simulink model "AEROATCSS"  (R2024b)
settings: Solver=ode45  StartTime=0.0  StopTime=10000  MaxStep=0.25  RelTol=1e-3
PreLoadFcn:
  | initialize_model_data;
  | appdesignparameteraeroatcss_exported_last1;
model workspace (MAT data in the model file):
  AZ_Sep = Simulink.Parameter
  AZ_Sep.Complexity = 'real'
  AZ_Sep.Dimensions = [0 0]
  AZ_Sep.DataType = 'auto'
  BwPw = Simulink.Parameter
  BwPw.Complexity = 'real'
  BwPw.Dimensions = [0 0]
  BwPw.DataType = 'auto'
  E = Simulink.Parameter
  E.Complexity = 'real'
  E.Dimensions = [0 0]
  E.DataType = 'auto'
  EL_Sep = Simulink.Parameter
  EL_Sep.Complexity = 'real'
  EL_Sep.Dimensions = [0 0]
  EL_Sep.DataType = 'auto'
  Lambda = Simulink.Parameter
  Lambda.Complexity = 'real'
  Lambda.Dimensions = [0 0]
  Lambda.DataType = 'auto'
  Loss = Simulink.Parameter
  Loss.Complexity = 'real'
  Loss.Dimensions = [0 0]
  Loss.DataType = 'auto'
  Noise = Simulink.Parameter
  Noise.Complexity = 'real'
  Noise.Dimensions = [0 0]
  Noise.DataType = 'auto'
  Pt = Simulink.Parameter
  Pt.Complexity = 'real'
  Pt.Dimensions = [0 0]
  Pt.DataType = 'auto'
  Rres = Simulink.Parameter
  Rres.Complexity = 'real'
  Rres.Dimensions = [0 0]
  Rres.DataType = 'auto'
  SNR = Simulink.Parameter
  SNR.Complexity = 'real'
  SNR.Dimensions = [0 0]
  SNR.DataType = 'auto'
  Temp = Simulink.Parameter
  Temp.Complexity = 'real'
  Temp.Dimensions = [0 0]
  Temp.DataType = 'auto'
  rainfall = Simulink.Parameter
  rainfall.Complexity = 'real'
  rainfall.Dimensions = [0 0]
  rainfall.DataType = 'auto'
values from neighbouring files (symbols this model uses):
  lambda_bp = [0.057, 0.075, 0.1, 0.15, 0.3]    [initialize_model_data.m]
  rainfall_bp = [0.0, 0.25, 1, 4, 16]    [initialize_model_data.m]
  sigma_table = [ ... (first row only)    [initialize_model_data.m]
settings Model: Creator=Sangam  LastModifiedBy=Sangam
settings DataIOCC: SaveFormat=Array  SaveOutput=off  SignalLogging=off  SaveTime=off  ReturnWorkspaceOutputs=off
settings DebuggingCC: MultiTaskCondExecSysMsg=none
settings ModelReferenceCC: EnableRefExpFcnMdlSchedulingChecks=on  PropagateSignalLabelsOutOfModel=off

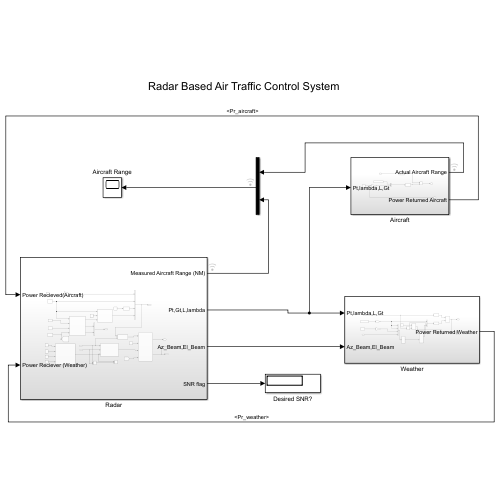
[thumbnail: Simulink's stored preview of the top-level diagram]
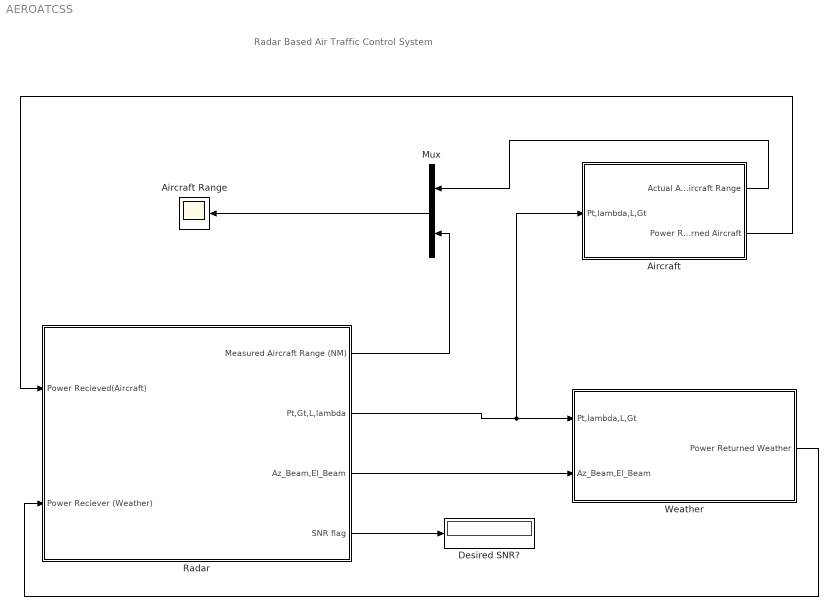
== system AEROATCSS ==
  note: Radar Based Air Traffic Control System
  Aircraft : Subsystem
  Aircraft Range : Scope
  Desired SNR? : Display
  Mux : Mux  Inputs=2
  Radar : Subsystem
  Weather : Subsystem
  wires:
  Radar/4(SNR flag) -> Desired SNR?/1
  Radar/1(Measured Aircraft Range (NM)) -> Mux/2
  Radar/2(Pt,Gt,L,lambda) -> Aircraft/1(Pt,lambda,L,Gt), Weather/1(Pt,lambda,L,Gt)
  Radar/3(Az_Beam,El_Beam) -> Weather/2(Az_Beam,El_Beam)
  Weather/1(Power Returned Weather) -> Radar/2("Power Reciever (Weather) ")
  Aircraft/1(Actual Aircraft Range) -> Mux/1
  Mux/1 -> Aircraft Range/1
  Aircraft/2(Power Returned Aircraft) -> Radar/1(Power Recieved(Aircraft))

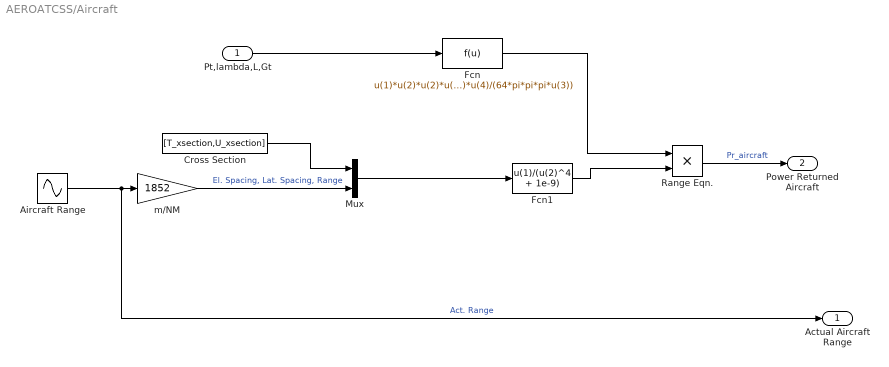
== system AEROATCSS/Aircraft ==
  Pt,lambda,L,Gt : Inport
  Aircraft Range : Sin  Amplitude=25  Bias=35  Frequency=0.0025  SampleTime=0
  Cross Section : FromWorkspace  VariableName=[T_xsection,U_xsection]  Interpolate=off  ZeroCross=off  OutputAfterFinalValue=Holding final value
  Fcn : Fcn  Expr=u(1)*u(2)*u(2)*u(4)*u(4)/(64*pi*pi*pi*u(3))
  Fcn1 : Fcn  Expr=u(1)/(u(2)^4 + 1e-9)
  Mux : Mux  Inputs=2
  Range Eqn. : Product  InputSameDT=on  RndMeth=Zero  SaturateOnIntegerOverflow=on  OutDataTypeStr=Inherit: Same as first input
  m/NM : Gain  Gain=1852
  Actual Aircraft Range : Outport
  Power Returned Aircraft : Outport  Port=2
  wires:
  Fcn1/1 -> Range Eqn./2
  Mux/1 -> Fcn1/1
  Aircraft Range/1 -> Actual Aircraft Range/1, m/NM/1  "Act. Range"
  m/NM/1 -> Mux/2  "El. Spacing, Lat. Spacing, Range"
  Pt,lambda,L,Gt/1 -> Fcn/1
  Range Eqn./1 -> Power Returned Aircraft/1  "Pr_aircraft"
  Cross Section/1 -> Mux/1
  Fcn/1 -> Range Eqn./1

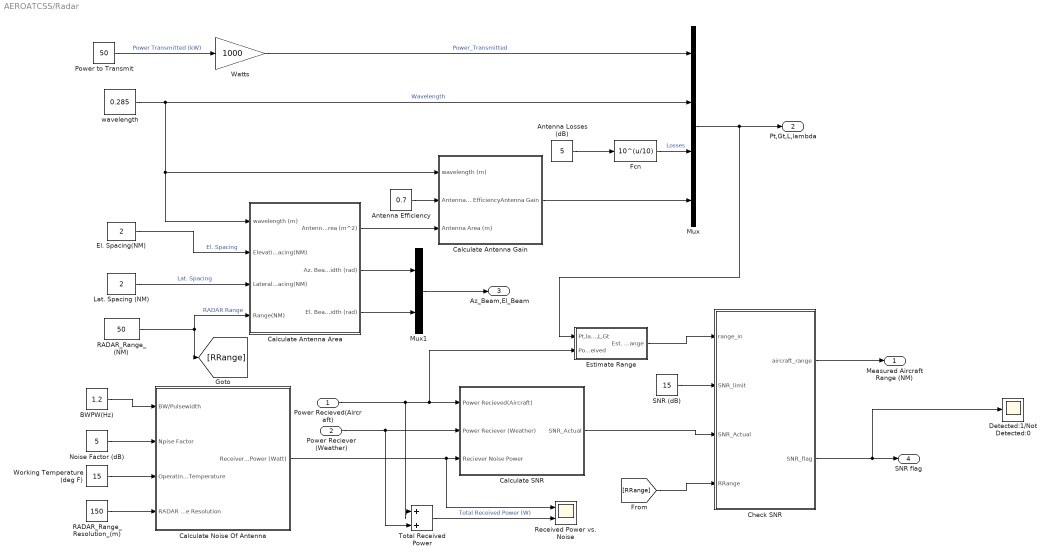
== system AEROATCSS/Radar ==
  Power Recieved(Aircraft) : Inport
  "Power Reciever (Weather) " : Inport  Port=2
  Antenna Efficiency : Constant  Value=0.7
  Antenna Losses (dB) : Constant  Value=5
  BWPW(Hz) : Constant  Value=1.2
  Calculate Antenna Area : Subsystem
  Calculate Antenna Gain : Subsystem
  Calculate Noise Of Antenna : Subsystem
  Calculate SNR : Subsystem
  Check SNR : Stateflow chart  TreatAsAtomicUnit=on
  Detected:1/Not Detected:0 : Scope
  El. Spacing(NM) : Constant  Value=2
  Estimate Range : Subsystem
  Fcn : Fcn  Expr=10^(u/10)
  Lat. Spacing (NM) : Constant  Value=2
  Mux : Mux
  Mux1 : Mux  Inputs=2
  Noise Factor (dB) : Constant  Value=5
  Power to Transmit : Constant  Value=50
  RADAR_Range_(NM) : Constant  Value=50
  RADAR_Range_Resolution_(m) : Constant  Value=150
  Received Power vs. Noise : Scope  NumInputPorts=2
  SNR (dB) : Constant  Value=15
  Total Received Power : Sum  Inputs=|++
  Watts : Gain  Gain=1000  SaturateOnIntegerOverflow=on  OutDataTypeStr=Inherit: Same as input  ParamDataTypeStr=Inherit: Same as input
  Working Temperature (deg F) : Constant  Value=15
  "wavelength " : Constant  Value=0.285
  Measured Aircraft Range (NM) : Outport
  Pt,Gt,L,lambda : Outport  Port=2
  Az_Beam,El_Beam : Outport  Port=3
  SNR flag : Outport  Port=4
  wires:
  Calculate Antenna Area/1(Antenna Area (m^2)) -> Calculate Antenna Gain/3(Antenna Area (m))
  Fcn/1 -> Mux/3  "Losses"
  Calculate Antenna Gain/1("Antenna Gain ") -> Mux/4
  Lat. Spacing (NM)/1 -> Calculate Antenna Area/3(Lateral Spacing(NM))  "Lat. Spacing"
  El. Spacing(NM)/1 -> Calculate Antenna Area/2(Elevation Spacing(NM))  "El. Spacing"
  "Power Reciever (Weather) "/1 -> Total Received Power/2, Calculate SNR/2("Power Reciever (Weather) ")
  Estimate Range/1(Est. Range) -> Check SNR/1(range_in)
  Antenna Losses (dB)/1 -> Fcn/1
  RADAR_Range_(NM)/1 -> Calculate Antenna Area/4(Range(NM)), [RRange]  "RADAR Range"
  "wavelength "/1 -> Calculate Antenna Gain/1(wavelength (m)), Calculate Antenna Area/1(wavelength (m)), Mux/2  "Wavelength"
  Power to Transmit/1 -> Watts/1  "Power Transmitted (kW)"
  Check SNR/1(aircraft_range) -> Measured Aircraft Range (NM)/1
  Working Temperature (deg F)/1 -> Calculate Noise Of Antenna/3(Operating Temperature)
  Calculate Noise Of Antenna/1(Receiver Noise Power (Watt)) -> Received Power vs. Noise/1, Calculate SNR/3(Reciever Noise Power)
  RADAR_Range_Resolution_(m)/1 -> Calculate Noise Of Antenna/4(RADAR Range Resolution)
  Mux1/1 -> Az_Beam,El_Beam/1
  Calculate SNR/1(SNR_Actual) -> Check SNR/3(SNR_Actual)
  Watts/1 -> Mux/1  "Power_Transmitted"
  Power Recieved(Aircraft)/1 -> Total Received Power/1, Estimate Range/2(Power Received), Calculate SNR/1(Power Recieved(Aircraft))
  SNR (dB)/1 -> Check SNR/2(SNR_limit)
  BWPW(Hz)/1 -> Calculate Noise Of Antenna/1(BW/Pulsewidth)
  Noise Factor (dB)/1 -> Calculate Noise Of Antenna/2(Npise Factor)
  Calculate Antenna Area/2(Az. Beamwidth (rad)) -> Mux1/1
  Calculate Antenna Area/3(El. Beamwidth (rad)) -> Mux1/2
  Antenna Efficiency/1 -> Calculate Antenna Gain/2(Antenna Efficiency)
  [RRange] -> Check SNR/4(RRange)
  Check SNR/2(SNR_flag) -> Detected:1/Not Detected:0/1, SNR flag/1
  Mux/1 -> Estimate Range/1(Pt,lambda,L,Gt), Pt,Gt,L,lambda/1
  Total Received Power/1 -> Received Power vs. Noise/2  "Total Received Power (W)"

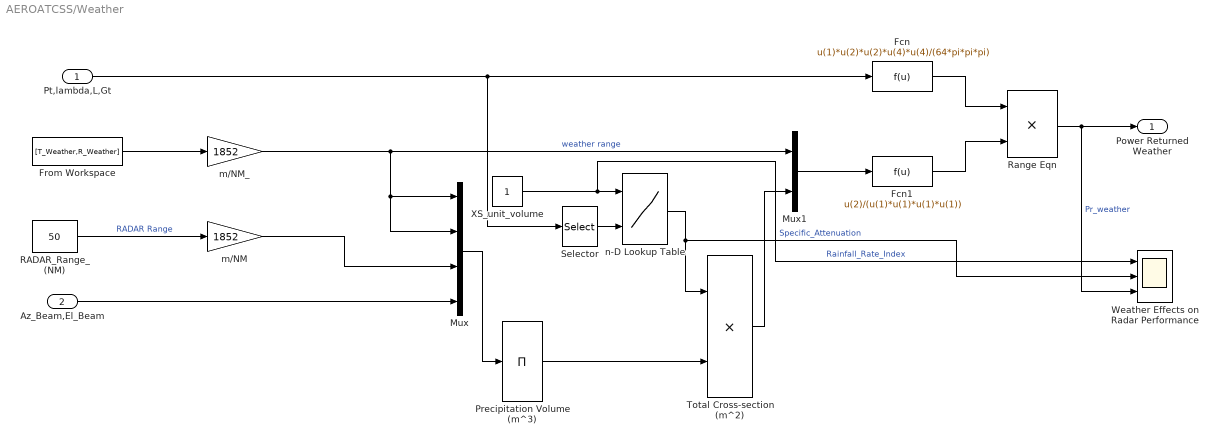
== system AEROATCSS/Weather ==
  Pt,lambda,L,Gt : Inport
  Az_Beam,El_Beam : Inport  Port=2
  Fcn : Fcn  Expr=u(1)*u(2)*u(2)*u(4)*u(4)/(64*pi*pi*pi)
  Fcn1 : Fcn  Expr=u(2)/(u(1)*u(1)*u(1)*u(1))
  From Workspace : FromWorkspace  VariableName=[T_Weather,R_Weather]  Interpolate=off  ZeroCross=off  OutputAfterFinalValue=Holding final value
  Mux : Mux
  Mux1 : Mux  Inputs=2
  Precipitation Volume (m^3) : Product  Inputs=*  InputSameDT=on  RndMeth=Zero  SaturateOnIntegerOverflow=on  OutDataTypeStr=Inherit: Same as first input
  RADAR_Range_(NM) : Constant  Value=50
  Range Eqn : Product  InputSameDT=on  RndMeth=Zero  SaturateOnIntegerOverflow=on  OutDataTypeStr=Inherit: Same as first input
  Selector : Selector  InputPortWidth=4  IndexOptions=Index vector (dialog)  Indices=2  OutputSizes=1
  Total Cross-section (m^2) : Product  InputSameDT=on  RndMeth=Zero  SaturateOnIntegerOverflow=on  OutDataTypeStr=Inherit: Same as first input
  Weather Effects on Radar Performance : Scope  NumInputPorts=3
  XS_unit_volume : Constant
  m/NM : Gain  Gain=1852  SaturateOnIntegerOverflow=on  OutDataTypeStr=Inherit: Same as input  ParamDataTypeStr=Inherit: Same as input
  m/NM_ : Gain  Gain=1852  SaturateOnIntegerOverflow=on  OutDataTypeStr=Inherit: Same as input  ParamDataTypeStr=Inherit: Same as input
  n-D Lookup Table : Lookup_n-D  BreakpointsForDimension1=rainfall_bp  BreakpointsForDimension2=lambda_bp  BreakpointsForDimension3=[5, 7]  Table=sigma_table  SaturateOnIntegerOverflow=on
      settings: InputPortMap=u0,u1
  Power Returned Weather : Outport
  wires:
  Selector/1 -> n-D Lookup Table/2
  Fcn/1 -> Range Eqn/1
  Pt,lambda,L,Gt/1 -> Selector/1, Fcn/1
  Az_Beam,El_Beam/1 -> Mux/4
  RADAR_Range_(NM)/1 -> m/NM/1  "RADAR Range"
  XS_unit_volume/1 -> Weather Effects on Radar Performance/1, n-D Lookup Table/1  "Rainfall_Rate_Index"
  From Workspace/1 -> m/NM_/1
  Total Cross-section (m^2)/1 -> Mux1/2
  m/NM/1 -> Mux/3
  Mux/1 -> Precipitation Volume (m^3)/1
  Fcn1/1 -> Range Eqn/2
  m/NM_/1 -> Mux/1, Mux/2, Mux1/1  "weather range"
  n-D Lookup Table/1 -> Weather Effects on Radar Performance/2, Total Cross-section (m^2)/1  "Specific_Attenuation"
  Range Eqn/1 -> Weather Effects on Radar Performance/3, Power Returned Weather/1  "Pr_weather"
  Mux1/1 -> Fcn1/1
  Precipitation Volume (m^3)/1 -> Total Cross-section (m^2)/2

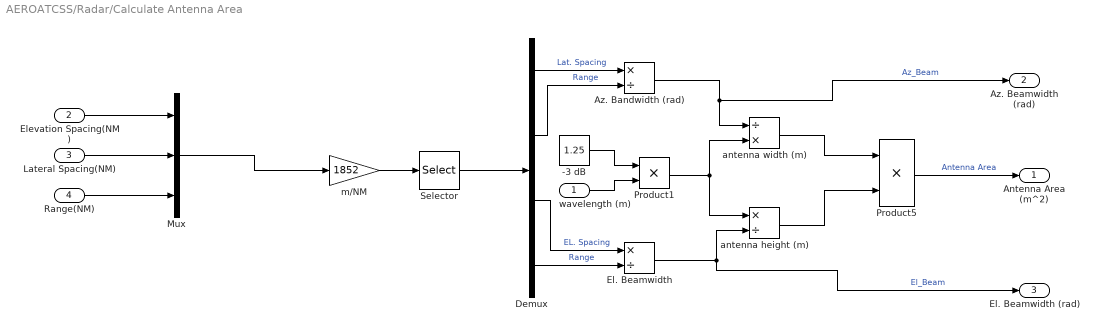
== system AEROATCSS/Radar/Calculate Antenna Area ==
  wavelength (m) : Inport
  Elevation Spacing(NM) : Inport  Port=2
  Lateral Spacing(NM) : Inport  Port=3
  Range(NM) : Inport  Port=4
  -3 dB : Constant  Value=1.25
  Az. Bandwidth (rad) : Product  Inputs=*/  InputSameDT=on  RndMeth=Zero  SaturateOnIntegerOverflow=on  OutDataTypeStr=Inherit: Same as first input
  Demux : Demux
  El. Beamwidth : Product  Inputs=*/  InputSameDT=on  RndMeth=Zero  SaturateOnIntegerOverflow=on  OutDataTypeStr=Inherit: Same as first input
  Mux : Mux  Inputs=3
  Product1 : Product  Inputs=**  InputSameDT=on  RndMeth=Zero  SaturateOnIntegerOverflow=on  OutDataTypeStr=Inherit: Same as first input
  Product5 : Product  InputSameDT=on  RndMeth=Zero  SaturateOnIntegerOverflow=on  OutDataTypeStr=Inherit: Same as first input
  Selector : Selector  InputPortWidth=3  IndexOptions=Index vector (dialog)  Indices=[1 3 2 3]  OutputSizes=1
  antenna height (m) : Product  Inputs=*/  InputSameDT=on  RndMeth=Zero  SaturateOnIntegerOverflow=on  OutDataTypeStr=Inherit: Same as first input
  antenna width (m) : Product  Inputs=/*  RndMeth=Zero  SaturateOnIntegerOverflow=on  OutDataTypeStr=Inherit: Same as first input
  m/NM : Gain  Gain=1852  SaturateOnIntegerOverflow=on  OutDataTypeStr=Inherit: Same as input  ParamDataTypeStr=Inherit: Same as input
  Antenna Area (m^2) : Outport
  Az. Beamwidth (rad) : Outport  Port=2
  El. Beamwidth (rad) : Outport  Port=3
  wires:
  Demux/1 -> Az. Bandwidth (rad)/1  "Lat. Spacing"
  Mux/1 -> m/NM/1
  Demux/2 -> Az. Bandwidth (rad)/2  "Range"
  Demux/4 -> El. Beamwidth/2  "Range"
  antenna height (m)/1 -> Product5/2
  Range(NM)/1 -> Mux/3
  -3 dB/1 -> Product1/1
  Selector/1 -> Demux/1
  Product1/1 -> antenna height (m)/1, antenna width (m)/2
  El. Beamwidth/1 -> El. Beamwidth (rad)/1, antenna height (m)/2  "El_Beam"
  wavelength (m)/1 -> Product1/2
  Product5/1 -> Antenna Area (m^2)/1  "Antenna Area"
  antenna width (m)/1 -> Product5/1
  Lateral Spacing(NM)/1 -> Mux/2
  Elevation Spacing(NM)/1 -> Mux/1
  Demux/3 -> El. Beamwidth/1  "EL. Spacing"
  m/NM/1 -> Selector/1
  Az. Bandwidth (rad)/1 -> antenna width (m)/1, Az. Beamwidth (rad)/1  "Az_Beam"

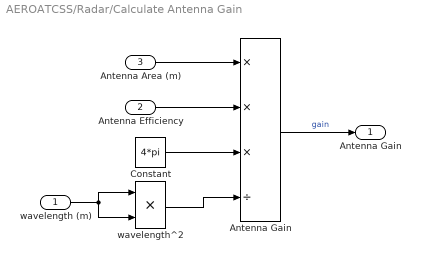
== system AEROATCSS/Radar/Calculate Antenna Gain ==
  wavelength (m) : Inport
  Antenna Efficiency : Inport  Port=2
  Antenna Area (m) : Inport  Port=3
  Antenna Gain : Product  Inputs=***/  InputSameDT=on  RndMeth=Zero  SaturateOnIntegerOverflow=on  OutDataTypeStr=Inherit: Same as first input
  Constant : Constant  Value=4*pi
  wavelength^2 : Product  InputSameDT=on  RndMeth=Zero  SaturateOnIntegerOverflow=on  OutDataTypeStr=Inherit: Same as first input
  "Antenna Gain " : Outport
  wires:
  Antenna Area (m)/1 -> Antenna Gain/1
  wavelength^2/1 -> Antenna Gain/4
  Constant/1 -> Antenna Gain/3
  wavelength (m)/1 -> wavelength^2/1, wavelength^2/2
  Antenna Gain/1 -> "Antenna Gain "/1  "gain"
  Antenna Efficiency/1 -> Antenna Gain/2

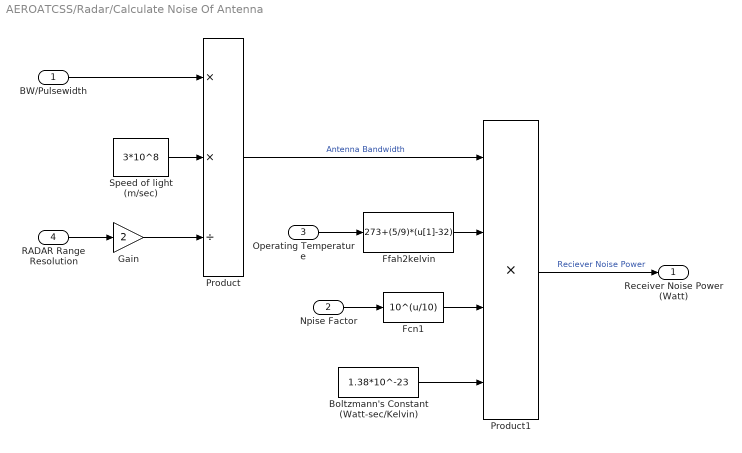
== system AEROATCSS/Radar/Calculate Noise Of Antenna ==
  BW/Pulsewidth : Inport
  Npise Factor : Inport  Port=2
  Operating Temperature : Inport  Port=3
  RADAR Range Resolution : Inport  Port=4
  Boltzmann's Constant (Watt-sec/Kelvin) : Constant  Value=1.38*10^-23
  Fcn1 : Fcn  Expr=10^(u/10)
  Ffah2kelvin : Fcn  Expr=273+(5/9)*(u[1]-32)
  Gain : Gain  Gain=2  ParamDataTypeStr=Inherit: Inherit from 'Gain'  SaturateOnIntegerOverflow=on  OutDataTypeStr=Inherit: Same as input
  Product : Product  Inputs=**/  InputSameDT=on  RndMeth=Zero  SaturateOnIntegerOverflow=on  OutDataTypeStr=Inherit: Same as first input
  Product1 : Product  Inputs=4  InputSameDT=on  SaturateOnIntegerOverflow=on  OutDataTypeStr=Inherit: Same as first input
  Speed of light (m/sec) : Constant  Value=3*10^8
  Receiver Noise Power (Watt) : Outport
  wires:
  Gain/1 -> Product/3
  Speed of light (m/sec)/1 -> Product/2
  Npise Factor/1 -> Fcn1/1
  Ffah2kelvin/1 -> Product1/2
  Product/1 -> Product1/1  "Antenna Bandwidth"
  BW/Pulsewidth/1 -> Product/1
  Operating Temperature/1 -> Ffah2kelvin/1
  RADAR Range Resolution/1 -> Gain/1
  Boltzmann's Constant (Watt-sec/Kelvin)/1 -> Product1/4
  Fcn1/1 -> Product1/3
  Product1/1 -> Receiver Noise Power (Watt)/1  "Reciever Noise Power"

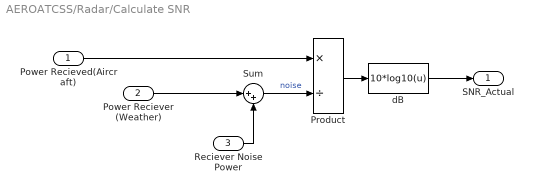
== system AEROATCSS/Radar/Calculate SNR ==
  Power Recieved(Aircraft) : Inport
  "Power Reciever (Weather) " : Inport  Port=2
  Reciever Noise Power : Inport  Port=3
  Product : Product  Inputs=*/  InputSameDT=on  RndMeth=Zero  SaturateOnIntegerOverflow=on  OutDataTypeStr=Inherit: Same as first input
  Sum : Sum  Inputs=|++  InputSameDT=on  SaturateOnIntegerOverflow=on  OutDataTypeStr=Inherit: Same as first input
  dB : Fcn  Expr=10*log10(u)
  SNR_Actual : Outport
  wires:
  "Power Reciever (Weather) "/1 -> Sum/1
  Reciever Noise Power/1 -> Sum/2
  dB/1 -> SNR_Actual/1
  Product/1 -> dB/1
  Sum/1 -> Product/2  "noise"
  Power Recieved(Aircraft)/1 -> Product/1

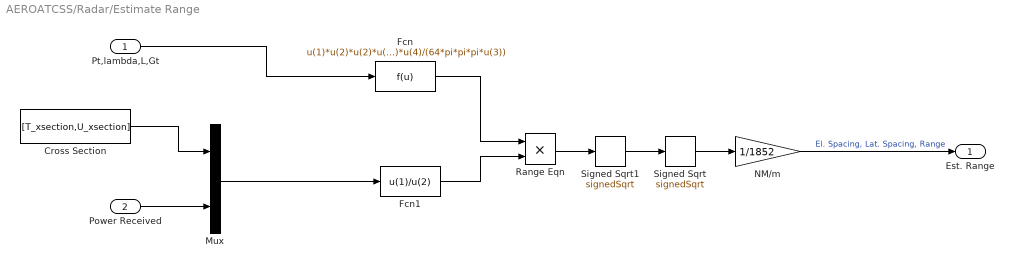
== system AEROATCSS/Radar/Estimate Range ==
  Pt,lambda,L,Gt : Inport
  Power Received : Inport  Port=2
  "Cross Section " : FromWorkspace  VariableName=[T_xsection,U_xsection]  ZeroCross=off
  Fcn : Fcn  Expr=u(1)*u(2)*u(2)*u(4)*u(4)/(64*pi*pi*pi*u(3))
  Fcn1 : Fcn  Expr=u(1)/u(2)
  Mux : Mux  Inputs=2
  NM/m : Gain  Gain=1/1852  SaturateOnIntegerOverflow=on  OutDataTypeStr=Inherit: Same as input  ParamDataTypeStr=Inherit: Same as input
  Range Eqn : Product  InputSameDT=on  RndMeth=Zero  SaturateOnIntegerOverflow=on  OutDataTypeStr=Inherit: Same as first input
  Signed Sqrt : Sqrt  Operator=signedSqrt
  Signed Sqrt1 : Sqrt  Operator=signedSqrt
  Est. Range : Outport
  wires:
  Fcn1/1 -> Range Eqn/2
  NM/m/1 -> Est. Range/1  "El. Spacing, Lat. Spacing, Range"
  "Cross Section "/1 -> Mux/1
  Signed Sqrt1/1 -> Signed Sqrt/1
  Power Received/1 -> Mux/2
  Pt,lambda,L,Gt/1 -> Fcn/1
  Signed Sqrt/1 -> NM/m/1
  Fcn/1 -> Range Eqn/1
  Mux/1 -> Fcn1/1
  Range Eqn/1 -> Signed Sqrt1/1

== stateflow chart AEROATCSS/Radar/Check SNR ==
  settings: updateMethod=CONTINUOUS
  state Visibility [parallel]
    settings: executionOrder=1
    state detect
      during: aircraft_range = range_in;
    state no_detect
      during: aircraft_range =0;
    (default) -> (junction 3)
    (junction 3) -> no_detect [order 1] : [(SNR_Actual <= 6) || (range_in > RRange)]{aircraft_range =0;}
    (junction 3) -> detect [order 2] : {aircraft_range = range_in;}%(SNR_Actual > 6) && (range_in <= RRange)
    detect -> no_detect : [(SNR_Actual <= 6) || (range_in > RRange)]{aircraft_range=0;}
    no_detect -> detect : [(SNR_Actual > 6) && (range_in <= RRange)]{aircraft_range = range_in;}
  state SNR [parallel]
    settings: executionOrder=2
    state Less_than
    state Equal_to_or_Greater_than
    (default) -> (junction 6)
    (junction 6) -> Equal_to_or_Greater_than [order 1] : [SNR_Actual>=SNR_limit]{SNR_flag=1;}
    (junction 6) -> Less_than [order 2] : {SNR_flag=0;}%(SNR_Actual > 6) && (range_in <= RRange)
    Equal_to_or_Greater_than -> Less_than : [SNR_Actual<SNR_limit]{SNR_flag=0;}
    Less_than -> Equal_to_or_Greater_than : [SNR_Actual>=SNR_limit]{SNR_flag=1;}
  data: aircraft_range output; range_in input; SNR_limit input; SNR_Actual input; RRange input; SNR_flag output
